simulink model "BufMinMax_tests"  (R2024a)
settings: Solver=VariableStepAuto  StartTime=0.0  StopTime=SIM_TIME  RelTol=1e-3
undefined symbols (not defined in the file or in its folder): BUFFER_LEN, SAMPLING_FREQ
settings Model: Creator=Jan Rosa  LastModifiedBy=Jan Rosa

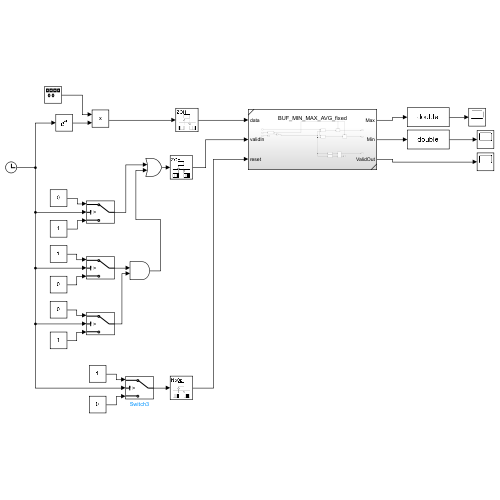
[thumbnail: Simulink's stored preview of the top-level diagram]
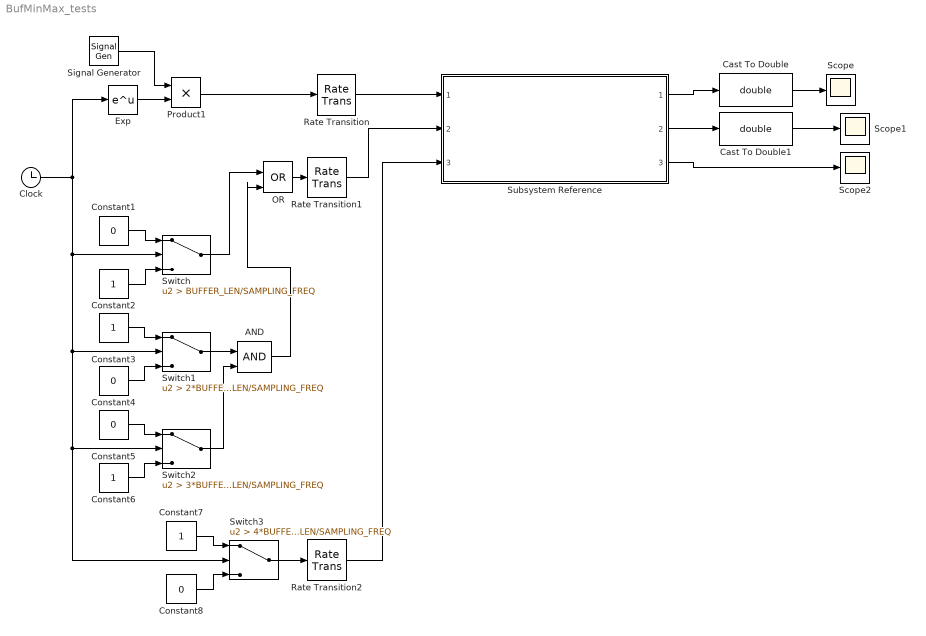
== system BufMinMax_tests ==
  AND : Logic  IconShape=distinctive  AllPortsSameDT=off  OutDataTypeStr=boolean
  Cast To Double : DataTypeConversion  OutDataTypeStr=double  SaturateOnIntegerOverflow=off  RndMeth=Floor
  Cast To Double1 : DataTypeConversion  OutDataTypeStr=double  SaturateOnIntegerOverflow=off  RndMeth=Floor
  Clock : Clock
  Constant{1,4..5,8} (4 alike) : Constant  Value=0
  Constant{2..3,6..7} (4 alike) : Constant
  Exp : Math
  OR : Logic  Operator=OR  IconShape=distinctive  AllPortsSameDT=off  OutDataTypeStr=boolean
  Product1 : Product  OutDataTypeStr=fixdt(1,12,11)
  Rate Transition : RateTransition  OutPortSampleTime=1/SAMPLING_FREQ
  Rate Transition1 : RateTransition  OutPortSampleTime=1/SAMPLING_FREQ
  Rate Transition2 : RateTransition  OutPortSampleTime=1/SAMPLING_FREQ
  Scope : Scope
  Scope1 : Scope
  Scope2 : Scope
  Signal Generator : SignalGenerator  Frequency=50
  Subsystem Reference : Subsystem  ReferencedSubsystem=BUF_MIN_MAX_AVG_fixed
  Switch : Switch  Criteria=u2 > Threshold  Threshold=BUFFER_LEN/SAMPLING_FREQ  SaturateOnIntegerOverflow=off  InputSameDT=off
  Switch1 : Switch  Criteria=u2 > Threshold  Threshold=2*BUFFER_LEN/SAMPLING_FREQ  SaturateOnIntegerOverflow=off  InputSameDT=off
  Switch2 : Switch  Criteria=u2 > Threshold  Threshold=3*BUFFER_LEN/SAMPLING_FREQ  SaturateOnIntegerOverflow=off  InputSameDT=off
  Switch3 : Switch  Criteria=u2 > Threshold  Threshold=4*BUFFER_LEN/SAMPLING_FREQ  OutDataTypeStr=boolean  SaturateOnIntegerOverflow=off  InputSameDT=off
  wires:
  Product1/1 -> Rate Transition/1
  Rate Transition/1 -> Subsystem Reference/1
  Switch/1 -> OR/1
  Switch3/1 -> Rate Transition2/1
  Subsystem Reference/1 -> Cast To Double/1
  Subsystem Reference/3 -> Scope2/1
  Subsystem Reference/2 -> Cast To Double1/1
  Exp/1 -> Product1/2
  Signal Generator/1 -> Product1/1
  Constant1/1 -> Switch/1
  Constant2/1 -> Switch/3
  Rate Transition1/1 -> Subsystem Reference/2
  Constant4/1 -> Switch1/3
  Constant3/1 -> Switch1/1
  OR/1 -> Rate Transition1/1
  Constant5/1 -> Switch2/1
  Constant6/1 -> Switch2/3
  Switch1/1 -> AND/1
  Switch2/1 -> AND/2
  AND/1 -> OR/2
  Clock/1 -> Exp/1, Switch2/2, Switch3/2, Switch1/2, Switch/2
  Constant8/1 -> Switch3/3
  Constant7/1 -> Switch3/1
  Rate Transition2/1 -> Subsystem Reference/3
  Cast To Double/1 -> Scope/1
  Cast To Double1/1 -> Scope1/1
